simulink model "regelNormalform2"  (Simulink 8.5)
settings: Solver=ode45  StartTime=0.0  StopTime=10.0  RelTol=1e-3
values from neighbouring files (symbols this model uses):
  n = length(pq1.p{:})    [RT_klausurvorb.m]    (also in regelNormalform_proc.m = [1 2 3])
  z = 8    [RT_ctrl_analyse_proc.m]    (also in RT_lead_lag_uebung.m = -40; regelNormalform_proc.m = [1 p 3])
settings Model: Creator=mainster  LastModifiedBy=mainster
settings DataIOCC: SignalLoggingSaveFormat=Dataset
settings OptimizationCC: ExpressionDepthLimit=128
settings DebuggingCC: UnderspecifiedInitializationDetection=Simplified  MergeDetectMultiDrivingBlocksExec=error  FcnCallInpInsideContextMsg=EnableAllAsError  StateNameClashWarn=none
settings GRTTargetCC: CombineOutputUpdateFcns=on  GRTInterface=off

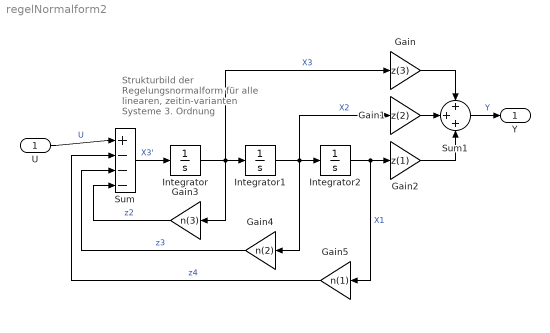
== system regelNormalform2 ==
  note: Strukturbild der Regelungsnormalform für alle linearen, zeitin-varianten Systeme 3. Ordnung
  U : Inport
  Gain : Gain  Gain=z(3)
  Gain1 : Gain  Gain=z(2)
  Gain2 : Gain  Gain=z(1)
  Gain3 : Gain  Gain=n(3)
  Gain4 : Gain  Gain=n(2)
  Gain5 : Gain  Gain=n(1)
  Integrator : Integrator
  Integrator1 : Integrator
  Integrator2 : Integrator
  Sum : Sum  Inputs=|+|---
  Sum1 : Sum  Inputs=+++
  Y : Outport
  wires:
  U/1 -> Sum/1  "U"
  Gain/1 -> Sum1/1
  Gain1/1 -> Sum1/2
  Gain2/1 -> Sum1/3
  Integrator/1 -> Gain3/1, Gain/1, Integrator1/1  "X3"
  Integrator1/1 -> Gain4/1, Gain1/1, Integrator2/1  "X2"
  Sum/1 -> Integrator/1  "X3'"
  Gain5/1 -> Sum/2  "z4"
  Gain4/1 -> Sum/3  "z3"
  Gain3/1 -> Sum/4  "z2"
  Integrator2/1 -> Gain2/1, Gain5/1  "X1"
  Sum1/1 -> Y/1  "Y"
